simulink model "HQEV_MiL_20160830_integrate_2010a"  (Simulink 7.5)
settings: Solver=FixedStepDiscrete  StartTime=0.0  StopTime=inf  FixedStep=0.01  RelTol=1e-3
PostLoadFcn:
  | , if any(exist('dsrtsu_mdlpostloadfcn', 'file') == [2, 3, 6]), try dsrtsu_mdlpostloadfcn('Execute', bdroot); catch fprintf('Error in PostLoadFcn (dsrtsu_mdlpostloadfcn) for model "%s":\n %s\n', bdroot, lasterr); end, end,
values from neighbouring files (symbols this model uses):
  Bat_C_Ah = 36    [parameter_V1.mat]
  Bat_ocv_xIndex = [5 10 20 30 40 50 60 70 80 90 95]    [parameter_V1.mat]
  Bat_ocv_z = [329 332 340 345 347 351 358 372 377 386 391]    [parameter_V1.mat]
  Bat_R_ohm_z = [4.41 3.46 1.57 1.07 0.76 0.63 0.55 0.44 0.41 0.4 0.4 3.14 ... (66 elements, 11x6)]    [parameter_V1.mat]
  Bat_SOC_Init = 90    [parameter_V1.mat]
  Env_hum_pct_Ambient = 30    [parameter_V1.mat]
  Env_Slope_deg = 0    [parameter_V1.mat]
  Env_Temp_degC_Ambient = 25    [parameter_V1.mat]
  Env_v_kmph_HWind = 0    [parameter_V1.mat]
  Reducer_F_i = 7.23    [parameter_V1.mat]
  Reducer_R_i = 7.23    [parameter_V1.mat]
  Veh =     [parameter_V1.mat]
  Veh_A_m2_Fr = 2.246    [parameter_V1.mat]
  Veh_F_Brake =     [parameter_V1.mat]
  Veh_fac_AirDrag = 0.326    [parameter_V1.mat]
  Veh_fac_WhDragFrict_0 = 0.011    [parameter_V1.mat]
  Veh_g_mps2_C = 9.81    [parameter_V1.mat]
  Veh_GainBrake =     [parameter_V1.mat]
  Veh_h_m_COGHigh = 0.5    [parameter_V1.mat]
  Veh_J_kgm2_Wh = 1.3635    [parameter_V1.mat]
  Veh_L_m_AxlBas = 2.63    [parameter_V1.mat]
  Veh_M_kg = 1427    [parameter_V1.mat]
  Veh_mu_Brake = 0.4    [parameter_V1.mat]
  Veh_mu_Tyre =     [parameter_V1.mat]
  Veh_num_FrictPair = 8    [parameter_V1.mat]
  Veh_pct_Brk = 70    [parameter_V1.mat]
  Veh_r_dyn =     [parameter_V1.mat]
  Veh_r_m_BrkDisk = 0.136    [parameter_V1.mat]
  Veh_rho_kgpm3_Air = 1.2258    [parameter_V1.mat]
undefined symbols (not defined in the file or in its folder): DiscIntNeverNeededParam, p_bool_False_M, p_bool_True_M
libraries: BaseOperationLib_Browser x38, simulink x14, DTQC_lib x1, ERR_lib x1, MQM_lib x1, PTCL_lib x1, PUD_lib x1, TQD_lib x1, TQR_lib x1, VMM_lib x1, ACCA_lib x1, BBCA_lib x1
(part 11 of 15)

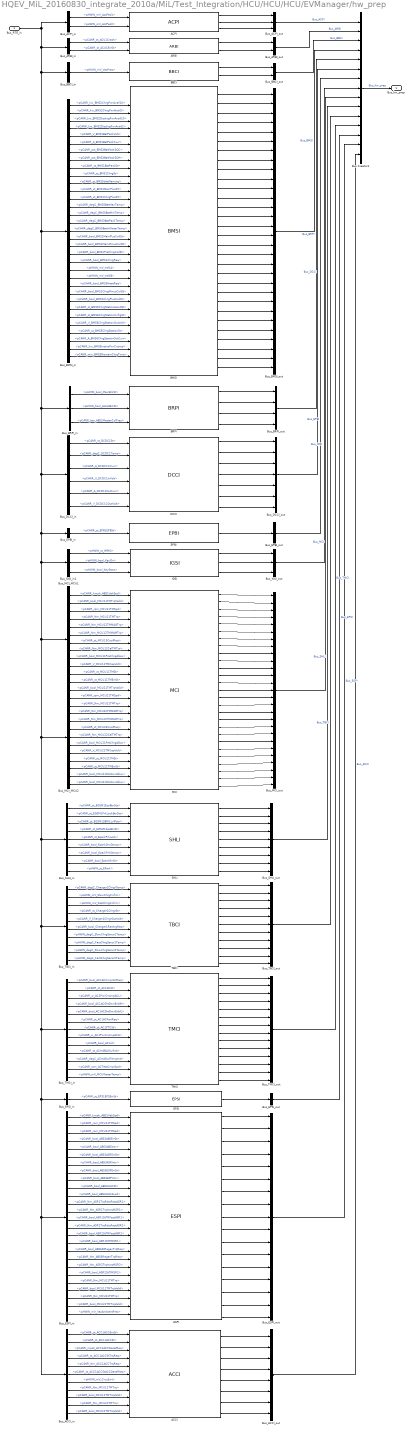
== system HQEV_MiL_20160830_integrate_2010a/MiL/Test_Integration/HCU/HCU/HCU/EVManager/hw_prep ==
  Bus_RTE_in : Inport  OutDataType=fixdt(1, 16)  OutScaling=2^0
  ACCI : ACCI_lib/ACCI  SystemSampleTime=-1
  ACPI : ACPI_lib/ACPI  SystemSampleTime=-1
  ARBI : ARBI_lib/ARBI  SystemSampleTime=-1
  BBCI : BBCI_lib/BBCI  SystemSampleTime=-1
  BMSI : BMSI_lib/BMSI  SystemSampleTime=-1
  BRPI : BRPI_lib/BRPI  SystemSampleTime=-1
  Bus Creator1 : BusCreator  Inputs=15
  Bus_ACCI_in : BusSelector  OutputSignals=pCANR_PT.pCANR_ACC1.pCANR_st_ACC1ACCErrSt,pCANR_PT.pCANR_ACC1.pCANR_st_ACC1ACCSt,pCANR_PT.pCANR_ACC1.pCANR_mps2_ACC1ACCDecelReq,pCANR_PT.pCANR_ACC1.pCANR_st_ACC1ACCStTrqReq,pCANR_PT.pCANR_ACC1.pCANR_Nm_ACC1ACCTrqReq,pCANR_PT.pCANR_ACC1.pCANR_st_ACC1ACCStACCDecelReq,IO.pHWIN_mV_CruzSwt,pCANR_EV.pCANR_MCU.pCANR_MCU1.pCANR_Nm_MCU11TMTrq,pCANR_EV.pCANR_MCU.pCANR_MCU1.pCANR_bool_MCU11TMTrqValid,pCANR_EV.pCANR_MCU.pCANR_MCU1.pCANR_Nm_MCU21TMTrq,pCANR_EV.pCANR_MCU.pCANR_MCU1.pCANR_bool_MCU21TMTrqValid
  Bus_ACCI_out : BusCreator  Inputs=8
  Bus_ACPI_in : BusSelector  OutputSignals=IO.pHWIN_mV_AccPed1,IO.pHWIN_mV_AccPed2
  Bus_ACPI_out : BusCreator  Inputs=3
  Bus_ARBI_in : BusSelector  OutputSignals=pCANR_PT.pCANR_Airbag1.pCANR_st_ACU1Crash,pCANR_PT.pCANR_Airbag1.pCANR_st_ACU1ErrSt
  Bus_ARBI_out : BusCreator  Inputs=2
  Bus_BBCI_in : BusSelector  OutputSignals=IO.pHWIN_mV_VacPres
  Bus_BBCI_out : BusCreator  Inputs=2
  Bus_BMSI_in : BusSelector  OutputSignals=pCANR_EV.pCANR_BMS.pCANR_BMS2.pCANR_kw_BMS2ChrgPwrAvail10,pCANR_EV.pCANR_BMS.pCANR_BMS2.pCANR_kw_BMS2ChrgPwrAvail2,pCANR_EV.pCANR_BMS.pCANR_BMS2.pCANR_kw_BMS2DischrgPwrAvail10,pCANR_EV.pCANR_BMS.pCANR_BMS2.pCANR_kw_BMS2DischrgPwrAvail2,pCANR_EV.pCANR_BMS.pCANR_BMS1.pCANR_V_BMS1BatPackVolt,pCANR_EV.pCANR_BMS.pCANR_BMS1.pCANR_A_BMS1BatPackCurr,pCANR_EV.pCANR_BMS.pCANR_BMS3.pCANR_pct_BMS3BatPackSOC,pCANR_EV.pCANR_BMS.pCANR_BMS3.pCANR_pct_BMS3BatPackSOH,pCANR_EV.pCANR_BMS.pCANR_BMS1.pCANR_st_BMS1BatPackSt,pCANR_EV.pCANR_BMS.pCANR_BMS1.pCANR_st_BMS1ChrgSt,pCANR_EV.pCANR_BMS.pCANR_BMS5.pCANR_st_BMS5IslaWarning,pCANR_EV.pCANR_BMS.pCANR_BMS1.pCANR_st_BMS1MainPlusFlt,pCANR_EV.pCANR_BMS.pCANR_BMS1.pCANR_st_BMS1ChrgPlusFlt,pCANR_EV.pCANR_BMS.pCANR_BMS4.pCANR_degC_BMS5BatMaxTemp,pCANR_EV.pCANR_BMS.pCANR_BMS4.pCANR_degC_BMS5BatMinTemp,pCANR_EV.pCANR_BMS.pCANR_BMS3.pCANR_degC_BMS3BatPackTemp,pCANR_EV.pCANR_BMS.pCANR_BMS4.pCANR_degC_BMS5BatInWaterTemp,pCANR_EV.pCANR_BMS.pCANR_BMS1.pCANR_bool_BMS1MainPlusCoilSt,pCANR_EV.pCANR_BMS.pCANR_BMS1.pCANR_bool_BMS1MainMinusCoilSt,pCANR_EV.pCANR_BMS.pCANR_BMS1.pCANR_bool_BMS1PreChrgCoilSt,pCANR_EV.pCANR_BMS.pCANR_BMS1.pCANR_bool_BMS1ChrgReq,IO.pHWIN_mV_IntlkA,IO.pHWIN_mV_IntlkB,pCANR_EV.pCANR_BMS.pCANR_BMS3.pCANR_bool_BMS3HeatReq,pCANR_EV.pCANR_BMS.pCANR_BMS1.pCANR_bool_BMS1ChrgMinusCoilSt,pCANR_EV.pCANR_BMS.pCANR_BMS1.pCANR_bool_BMS1ChrgPlusCoilSt,pCANR_EV.pCANR_BMS.pCANR_BMS5.pCANR_st_BMS5ChrgStationHandSt,pCANR_EV.pCANR_BMS.pCANR_BMS5.pCANR_st_BMS6ChrgStationCnfigSt,pCANR_EV.pCANR_BMS.pCANR_BMS5.pCANR_V_BMS6ChrgStationOutVolt,pCANR_EV.pCANR_BMS.pCANR_BMS5.pCANR_st_BMS5ChrgStationSt,pCANR_EV.pCANR_BMS.pCANR_BMS5.pCANR_A_BMS6ChrgStationOutCurr,pCANR_EV.pCANR_BMS.pCANR_BMS5.pCANR_kw_BMS6InstnsPwrCnsmp,pCANR_EV.pCANR_BMS.pCANR_BMS5.pCANR_min_BMS5RemainChrgTime
  Bus_BMSI_out : BusCreator  Inputs=30
  Bus_BRPI_in : BusSelector  OutputSignals=IO.pHWIN_bool_MainBrkSt,IO.pHWIN_bool_AssistBrkSt,pCANR_PT.pCANR_ABS.pCANR_ABS2.pCANR_bar_ABS2MasterCylPres
  Bus_BRPI_out : BusCreator
  Bus_DCCI_in : BusSelector  OutputSignals=pCANR_EV.pCANR_DCDC1.pCANR_st_DCDC1St,pCANR_EV.pCANR_DCDC1.pCANR_degC_DCDC1Temp,pCANR_EV.pCANR_DCDC1.pCANR_A_DCDC1InCurr,pCANR_EV.pCANR_DCDC1.pCANR_V_DCDC1InVolt,pCANR_EV.pCANR_DCDC1.pCANR_A_DCDC1OutCurr,pCANR_EV.pCANR_DCDC1.pCANR_V_DCDC1COutVolt
  Bus_DCCI_out : BusCreator  Inputs=7
  Bus_EPBI_in : BusSelector  OutputSignals=pCANR_PT.pCANR_EPB.pCANR_st_EPB1EPBSt
  Bus_EPBI_out : BusCreator  Inputs=1
  Bus_EPSI_in : BusSelector  OutputSignals=pCANR_PT.pCANR_ESP.pCANR_EPS1.pCANR_st_EPS1EPSErrSt
  Bus_EPSI_out : BusCreator  Inputs=1
  Bus_ESPI_in : BusSelector  OutputSignals=pCANR_PT.pCANR_ABS.pCANR_ABS1.pCANR_kmph_ABS1VehSpd,pCANR_EV.pCANR_MCU.pCANR_MCU1.pCANR_rpm_MCU11TMSpd,pCANR_EV.pCANR_MCU.pCANR_MCU1.pCANR_rpm_MCU21TMSpd,pCANR_PT.pCANR_ABS.pCANR_ABS3.pCANR_bool_ABS3ABSErrSt,pCANR_PT.pCANR_ABS.pCANR_ABS3.pCANR_bool_ABS3ABSIntv,pCANR_PT.pCANR_ABS.pCANR_ABS3.pCANR_bool_ABS3ASRErrSt,pCANR_PT.pCANR_ABS.pCANR_ABS3.pCANR_bool_ABS3ASRIntv,pCANR_PT.pCANR_ABS.pCANR_ABS3.pCANR_bool_ABS3ESPErrSt,pCANR_PT.pCANR_ABS.pCANR_ABS3.pCANR_bool_ABS3ESPIntv,pCANR_PT.pCANR_ABS.pCANR_ABS3.pCANR_bool_ABS3HHCSt,pCANR_PT.pCANR_ABS.pCANR_ABS3.pCANR_bool_ABS3HHCAvail,pCANR_PT.pCANR_ASR1.pCANR_Nm_ASR1TrqRdctFastASR1,pCANR_PT.pCANR_ASR1.pCANR_Nm_ASR1TrqIncrsMSR1,pCANR_PT.pCANR_ASR1.pCANR_bool_ASR1StTRFastASR1,pCANR_PT.pCANR_ASR2.pCANR_Nm_ASR2TrqRdctFastASR2,pCANR_PT.pCANR_ASR2.pCANR_bool_ASR2StTRFastASR2,pCANR_PT.pCANR_ASR1.pCANR_bool_ASR1StTIMSR1,pCANR_PT.pCANR_ABS6.pCANR_bool_ABS6StRegenTrqReq,pCANR_PT.pCANR_ABS6.pCANR_Nm_ABS6RegenTrqReq,pCANR_PT.pCANR_ASR2.pCANR_Nm_ASR2TrqIncrsMSR2,pCANR_PT.pCANR_ASR2.pCANR_bool_ASR2StTIMSR2,pCANR_EV.pCANR_MCU.pCANR_MCU1.pCANR_Nm_MCU11TMTrq,pCANR_EV.pCANR_MCU.pCANR_MCU1.pCANR_bool_MCU11TMTrqValid,pCANR_EV.pCANR_MCU.pCANR_MCU1.pCANR_Nm_MCU21TMTrq,pCANR_EV.pCANR_MCU.pCANR_MCU1.pCANR_bool_MCU21TMTrqValid,IO.pHWIN_mV_VacAmbientPres
  Bus_ESPI_out : BusCreator  Inputs=17
  Bus_IGSI_in1 : BusSelector  OutputSignals=IO.pHWIN_st_IMMO,IO.pHWIN_bool_KeyOn,IO.pHWIN_bool_KeyStart
  Bus_IGSI_out : BusCreator  Inputs=3
  Bus_MCI_MCU1 : BusSelector  OutputSignals=pCANR_PT.pCANR_ABS.pCANR_ABS1.pCANR_kmph_ABS1VehSpd,pCANR_EV.pCANR_MCU.pCANR_MCU1.pCANR_bool_MCU11TMTrqValid,pCANR_EV.pCANR_MCU.pCANR_MCU1.pCANR_rpm_MCU11TMSpd,pCANR_EV.pCANR_MCU.pCANR_MCU1.pCANR_Nm_MCU11TMTrq,pCANR_EV.pCANR_MCU.pCANR_MCU2.pCANR_Nm_MCU12TMMAGTrq,pCANR_EV.pCANR_MCU.pCANR_MCU2.pCANR_Nm_MCU12TMMAMTrq,pCANR_EV.pCANR_MCU.pCANR_MCU3.pCANR_st_MCU13CoolReq,pCANR_EV.pCANR_MCU.pCANR_MCU2.pCANR_Nm_MCU12CalTMTrq,pCANR_EV.pCANR_MCU.pCANR_MCU1.pCANR_bool_MCU11PreChrgAllow,pCANR_EV.pCANR_MCU.pCANR_MCU1.pCANR_V_MCU11TMCapVolt,pCANR_EV.pCANR_MCU.pCANR_MCU1.pCANR_st_MCU11TMSt,pCANR_EV.pCANR_MCU.pCANR_MCU1.pCANR_st_MCU11TMErrSt
  Bus_MCI_MCU2 : BusSelector  OutputSignals=pCANR_EV.pCANR_MCU.pCANR_MCU1.pCANR_bool_MCU21TMTrqValid,pCANR_EV.pCANR_MCU.pCANR_MCU1.pCANR_rpm_MCU21TMSpd,pCANR_EV.pCANR_MCU.pCANR_MCU1.pCANR_Nm_MCU21TMTrq,pCANR_EV.pCANR_MCU.pCANR_MCU2.pCANR_Nm_MCU22TMMAGTrq,pCANR_EV.pCANR_MCU.pCANR_MCU2.pCANR_Nm_MCU22TMMAMTrq,pCANR_EV.pCANR_MCU.pCANR_MCU3.pCANR_st_MCU23CoolReq,pCANR_EV.pCANR_MCU.pCANR_MCU2.pCANR_Nm_MCU22CalTMTrq,pCANR_EV.pCANR_MCU.pCANR_MCU1.pCANR_bool_MCU21PreChrgAllow,pCANR_EV.pCANR_MCU.pCANR_MCU1.pCANR_V_MCU21TMCapVolt,pCANR_EV.pCANR_MCU.pCANR_MCU1.pCANR_st_MCU21TMSt,pCANR_EV.pCANR_MCU.pCANR_MCU1.pCANR_st_MCU21TMErrSt,pCANR_EV.pCANR_MCU.pCANR_MCU1.pCANR_bool_MCU11ShtdwnAllow,pCANR_EV.pCANR_MCU.pCANR_MCU1.pCANR_bool_MCU21ShtdwnAllow
  Bus_MCI_out : BusCreator  Inputs=27
  Bus_SHLI_in : BusSelector  OutputSignals=pCANR_PT.pCANR_EGSM1.pCANR_st_EGSM1EcoBtnSts,pCANR_PT.pCANR_EGSM1.pCANR_st_EGSM1PrkLockBtnSts,pCANR_PT.pCANR_EGSM1.pCANR_st_EGSM1SBW1LvlPstn,pCANR_PT.pCANR_EGSM1.pCANR_st_EGSM1SecBtnSt,pCANR_PT.pCAN_ePark_STATE.pCANR_st_EparkPrkLock,pCANR_PT.pCAN_ePark_STATE.pCANR_bool_EparkDrvSensor,pCANR_PT.pCAN_ePark_STATE.pCANR_bool_EparkPrkSensor,pCANR_PT.pCAN_ePark_STATE.pCANR_bool_EparkErrSt,IO.pHWIN_st_EPark
  Bus_SHLI_out : BusCreator  Inputs=9
  Bus_TBCI_in : BusSelector  OutputSignals=pCANR_EV.pCANR_Charger1.pCANR_degC_Charger1ChrgrTemp,IO.pHWIN_mV_SlowChrgCnfrm,IO.pHWIN_mV_FastChrgCnfrm,pCANR_EV.pCANR_Charger1.pCANR_st_Charger1ChrgrSt,pCANR_EV.pCANR_Charger1.pCANR_V_Charger1ChrgrOutVolt,pCANR_EV.pCANR_Charger1.pCANR_bool_Charger1RechrgReq,IO.pHWIN_degC_SlowChrgSensr1Temp,IO.pHWIN_degC_FastChrgSensr1Temp,IO.pHWIN_degC_SlowChrgSensr2Temp,IO.pHWIN_degC_FastChrgSensr2Temp
  Bus_TBCI_out : BusCreator  Inputs=11
  Bus_TMCI_in : BusSelector  OutputSignals=pCANR_PT.pCANR_AC.pCANR_AC1.pCANR_bool_AC1ACCmprOnReq,pCANR_PT.pCANR_AC.pCANR_AC1.pCANR_st_AC1ACSt,pCANR_PT.pCANR_AC.pCANR_AC1.pCANR_w_AC1PwrCnsmpACL,pCANR_PT.pCANR_AC.pCANR_AC1.pCANR_bool_AC1ACShtDwnEnblH,pCANR_PT.pCANR_AC.pCANR_AC1.pCANR_bool_AC1ACShtDwnEnblL,pCANR_PT.pCANR_AC.pCANR_AC1.pCANR_st_AC1ACFanReq,pCANR_PT.pCANR_AC.pCANR_AC1.pCANR_st_AC1PTCSt,pCANR_PT.pCANR_AC.pCANR_AC1.pCANR_w_AC1PwrCnsmpACH,pCANR_PT.pCANR_AC.pCANR_AC1Indication.pCANR_bool_ACInd,pCANR_PT.pCANR_AC.pCANR_AC1Indication.pCANR_st_ACIndBLWLvlInd,pCANR_PT.pCANR_AC.pCANR_AC1Indication.pCANR_degC_ACIndOutTempInd,pCANR_PT.pCANR_AC.pCANR_ACTest.pCANR_rpm_ACTestCmprSpd,IO.pHWIN_mV_MCUWaterTemp
  Bus_TMCI_out : BusCreator  Inputs=14
  DCCI : DCCI_lib/DCCI  SystemSampleTime=-1
  EPBI : EPBI_lib/EPBI  SystemSampleTime=-1
  EPSI : EPSI_lib/EPSI  SystemSampleTime=-1
  ESPI : ESPI_lib/ESPI  SystemSampleTime=-1
  IGSI : IGSI_lib/IGSI  SystemSampleTime=-1
  MCI : MCI_lib/MCI  SystemSampleTime=-1
  SHLI : SHLI_lib/SHLI  SystemSampleTime=-1
  TBCI : TBCI_lib/TBCI  SystemSampleTime=-1
  TMCI : TMCI_lib/TMCI  SystemSampleTime=-1
  Bus_hw_prep : Outport  OutDataType=fixdt(1, 16)  OutScaling=2^0
  wires:
  TBCI/11 -> Bus_TBCI_out/11
  Bus_SHLI_in/8 -> SHLI/8  "<pCANR_bool_EparkErrSt>"
  TBCI/10 -> Bus_TBCI_out/10
  TBCI/9 -> Bus_TBCI_out/9
  TBCI/8 -> Bus_TBCI_out/8
  TBCI/7 -> Bus_TBCI_out/7
  TBCI/6 -> Bus_TBCI_out/6
  TBCI/5 -> Bus_TBCI_out/5
  TBCI/4 -> Bus_TBCI_out/4
  TBCI/3 -> Bus_TBCI_out/3
  TBCI/2 -> Bus_TBCI_out/2
  TBCI/1 -> Bus_TBCI_out/1
  TMCI/14 -> Bus_TMCI_out/14
  TMCI/13 -> Bus_TMCI_out/13
  TMCI/12 -> Bus_TMCI_out/12
  TMCI/11 -> Bus_TMCI_out/11
  TMCI/10 -> Bus_TMCI_out/10
  TMCI/9 -> Bus_TMCI_out/9
  TMCI/8 -> Bus_TMCI_out/8
  TMCI/7 -> Bus_TMCI_out/7
  TMCI/6 -> Bus_TMCI_out/6
  TMCI/5 -> Bus_TMCI_out/5
  TMCI/4 -> Bus_TMCI_out/4
  TMCI/3 -> Bus_TMCI_out/3
  TMCI/2 -> Bus_TMCI_out/2
  TMCI/1 -> Bus_TMCI_out/1
  Bus_TMCI_in/12 -> TMCI/12  "<pCANR_rpm_ACTestCmprSpd>"
  Bus_TMCI_in/13 -> TMCI/13  "<pHWIN_mV_MCUWaterTemp>"
  Bus_TMCI_in/11 -> TMCI/11  "<pCANR_degC_ACIndOutTempInd>"
  Bus_TMCI_in/10 -> TMCI/10  "<pCANR_st_ACIndBLWLvlInd>"
  Bus_TMCI_in/9 -> TMCI/9  "<pCANR_bool_ACInd>"
  Bus_TMCI_in/8 -> TMCI/8  "<pCANR_w_AC1PwrCnsmpACH>"
  Bus_TMCI_in/7 -> TMCI/7  "<pCANR_st_AC1PTCSt>"
  Bus_TMCI_in/6 -> TMCI/6  "<pCANR_st_AC1ACFanReq>"
  Bus_TMCI_in/5 -> TMCI/5  "<pCANR_bool_AC1ACShtDwnEnblL>"
  Bus_TMCI_in/4 -> TMCI/4  "<pCANR_bool_AC1ACShtDwnEnblH>"
  Bus_TMCI_in/3 -> TMCI/3  "<pCANR_w_AC1PwrCnsmpACL>"
  Bus_TMCI_in/2 -> TMCI/2  "<pCANR_st_AC1ACSt>"
  Bus_TMCI_in/1 -> TMCI/1  "<pCANR_bool_AC1ACCmprOnReq>"
  Bus_TMCI_out/1 -> Bus Creator1/12  "Bus_TMCI"
  DCCI/7 -> Bus_DCCI_out/7
  DCCI/6 -> Bus_DCCI_out/6
  DCCI/5 -> Bus_DCCI_out/5
  DCCI/4 -> Bus_DCCI_out/4
  DCCI/3 -> Bus_DCCI_out/3
  DCCI/2 -> Bus_DCCI_out/2
  DCCI/1 -> Bus_DCCI_out/1
  Bus_DCCI_in/6 -> DCCI/6  "<pCANR_V_DCDC1COutVolt>"
  Bus_DCCI_in/5 -> DCCI/5  "<pCANR_A_DCDC1OutCurr>"
  Bus_DCCI_in/4 -> DCCI/4  "<pCANR_V_DCDC1InVolt>"
  Bus_DCCI_in/3 -> DCCI/3  "<pCANR_A_DCDC1InCurr>"
  Bus_DCCI_in/2 -> DCCI/2  "<pCANR_degC_DCDC1Temp>"
  Bus_DCCI_in/1 -> DCCI/1  "<pCANR_st_DCDC1St>"
  Bus_DCCI_out/1 -> Bus Creator1/6  "Bus_DCCI"
  BMSI/30 -> Bus_BMSI_out/30
  BMSI/29 -> Bus_BMSI_out/29
  BMSI/28 -> Bus_BMSI_out/28
  BMSI/27 -> Bus_BMSI_out/27
  BMSI/26 -> Bus_BMSI_out/26
  BMSI/25 -> Bus_BMSI_out/25
  BMSI/24 -> Bus_BMSI_out/24
  BMSI/23 -> Bus_BMSI_out/23
  BMSI/22 -> Bus_BMSI_out/22
  BMSI/21 -> Bus_BMSI_out/21
  BMSI/20 -> Bus_BMSI_out/20
  BMSI/19 -> Bus_BMSI_out/19
  BMSI/18 -> Bus_BMSI_out/18
  BMSI/17 -> Bus_BMSI_out/17
  BMSI/16 -> Bus_BMSI_out/16
  BMSI/15 -> Bus_BMSI_out/15
  BMSI/14 -> Bus_BMSI_out/14
  BMSI/13 -> Bus_BMSI_out/13
  BMSI/12 -> Bus_BMSI_out/12
  Bus_SHLI_in/9 -> SHLI/9  "<pHWIN_st_EPark>"
  SHLI/9 -> Bus_SHLI_out/9
  SHLI/8 -> Bus_SHLI_out/8
  SHLI/7 -> Bus_SHLI_out/7
  SHLI/6 -> Bus_SHLI_out/6
  SHLI/5 -> Bus_SHLI_out/5
  SHLI/4 -> Bus_SHLI_out/4
  SHLI/3 -> Bus_SHLI_out/3
  SHLI/2 -> Bus_SHLI_out/2
  SHLI/1 -> Bus_SHLI_out/1
  Bus_SHLI_in/4 -> SHLI/4  "<pCANR_st_EGSM1SecBtnSt>"
  Bus_SHLI_in/7 -> SHLI/7  "<pCANR_bool_EparkPrkSensor>"
  Bus_SHLI_in/6 -> SHLI/6  "<pCANR_bool_EparkDrvSensor>"
  Bus_SHLI_in/5 -> SHLI/5  "<pCANR_st_EparkPrkLock>"
  Bus_SHLI_in/3 -> SHLI/3  "<pCANR_st_EGSM1SBW1LvlPstn>"
  Bus_SHLI_in/2 -> SHLI/2  "<pCANR_st_EGSM1PrkLockBtnSts>"
  Bus_SHLI_in/1 -> SHLI/1  "<pCANR_st_EGSM1EcoBtnSts>"
  BMSI/11 -> Bus_BMSI_out/11
  BMSI/10 -> Bus_BMSI_out/10
  BMSI/9 -> Bus_BMSI_out/9
  BMSI/8 -> Bus_BMSI_out/8
  BMSI/7 -> Bus_BMSI_out/7
  BMSI/6 -> Bus_BMSI_out/6
  BMSI/5 -> Bus_BMSI_out/5
  BMSI/4 -> Bus_BMSI_out/4
  BMSI/3 -> Bus_BMSI_out/3
  BMSI/2 -> Bus_BMSI_out/2
  BMSI/1 -> Bus_BMSI_out/1
  Bus_BMSI_in/13 -> BMSI/13  "<pCANR_st_BMS1ChrgPlusFlt>"
  Bus_BMSI_in/12 -> BMSI/12  "<pCANR_st_BMS1MainPlusFlt>"
  Bus_BMSI_in/33 -> BMSI/33  "<pCANR_min_BMS5RemainChrgTime>"
  Bus_ESPI_out/1 -> Bus Creator1/14  "Bus_ESPI"
  Bus_BMSI_in/32 -> BMSI/32  "<pCANR_kw_BMS6InstnsPwrCnsmp>"
  Bus_TBCI_in/10 -> TBCI/10  "<pHWIN_degC_FastChrgSensr2Temp>"
  Bus_TBCI_in/9 -> TBCI/9  "<pHWIN_degC_SlowChrgSensr2Temp>"
  Bus_TBCI_in/8 -> TBCI/8  "<pHWIN_degC_FastChrgSensr1Temp>"
  Bus_TBCI_in/7 -> TBCI/7  "<pHWIN_degC_SlowChrgSensr1Temp>"
  Bus_BMSI_in/1 -> BMSI/1  "<pCANR_kw_BMS2ChrgPwrAvail10>"
  Bus_IGSI_in1/3 -> IGSI/3  "<pHWIN_bool_KeyStart>"
  Bus_IGSI_in1/2 -> IGSI/2  "<pHWIN_bool_KeyOn>"
  Bus_IGSI_in1/1 -> IGSI/1  "<pHWIN_st_IMMO>"
  Bus_BMSI_in/31 -> BMSI/31  "<pCANR_A_BMS6ChrgStationOutCurr>"
  Bus_BMSI_in/30 -> BMSI/30  "<pCANR_st_BMS5ChrgStationSt>"
  Bus_BMSI_in/29 -> BMSI/29  "<pCANR_V_BMS6ChrgStationOutVolt>"
  Bus_BMSI_in/28 -> BMSI/28  "<pCANR_st_BMS6ChrgStationCnfigSt>"
  Bus_BMSI_in/27 -> BMSI/27  "<pCANR_st_BMS5ChrgStationHandSt>"
  Bus_BMSI_in/26 -> BMSI/26  "<pCANR_bool_BMS1ChrgPlusCoilSt>"
  Bus_BMSI_in/25 -> BMSI/25  "<pCANR_bool_BMS1ChrgMinusCoilSt>"
  Bus_BMSI_in/24 -> BMSI/24  "<pCANR_bool_BMS3HeatReq>"
  Bus_BMSI_in/23 -> BMSI/23  "<pHWIN_mV_IntlkB>"
  Bus_BMSI_in/22 -> BMSI/22  "<pHWIN_mV_IntlkA>"
  Bus_BMSI_in/21 -> BMSI/21  "<pCANR_bool_BMS1ChrgReq>"
  Bus_BMSI_in/20 -> BMSI/20  "<pCANR_bool_BMS1PreChrgCoilSt>"
  Bus_BMSI_in/19 -> BMSI/19  "<pCANR_bool_BMS1MainMinusCoilSt>"
  Bus_BMSI_in/18 -> BMSI/18  "<pCANR_bool_BMS1MainPlusCoilSt>"
  Bus_BMSI_in/17 -> BMSI/17  "<pCANR_degC_BMS5BatInWaterTemp>"
  Bus_BMSI_in/16 -> BMSI/16  "<pCANR_degC_BMS3BatPackTemp>"
  Bus_BMSI_in/15 -> BMSI/15  "<pCANR_degC_BMS5BatMinTemp>"
  Bus_BMSI_in/14 -> BMSI/14  "<pCANR_degC_BMS5BatMaxTemp>"
  Bus_BMSI_in/11 -> BMSI/11  "<pCANR_st_BMS5IslaWarning>"
  Bus_BMSI_in/10 -> BMSI/10  "<pCANR_st_BMS1ChrgSt>"
  Bus_BMSI_in/9 -> BMSI/9  "<pCANR_st_BMS1BatPackSt>"
  Bus_BMSI_in/8 -> BMSI/8  "<pCANR_pct_BMS3BatPackSOH>"
  Bus_BMSI_in/7 -> BMSI/7  "<pCANR_pct_BMS3BatPackSOC>"
  Bus_BMSI_in/6 -> BMSI/6  "<pCANR_A_BMS1BatPackCurr>"
  Bus_BMSI_in/5 -> BMSI/5  "<pCANR_V_BMS1BatPackVolt>"
  Bus_BMSI_in/4 -> BMSI/4  "<pCANR_kw_BMS2DischrgPwrAvail2>"
  Bus_BMSI_in/3 -> BMSI/3  "<pCANR_kw_BMS2DischrgPwrAvail10>"
  Bus_BMSI_in/2 -> BMSI/2  "<pCANR_kw_BMS2ChrgPwrAvail2>"
  IGSI/2 -> Bus_IGSI_out/2
  IGSI/1 -> Bus_IGSI_out/1
  BRPI/2 -> Bus_BRPI_out/2
  BRPI/1 -> Bus_BRPI_out/1
  Bus_BRPI_in/3 -> BRPI/3  "<pCANR_bar_ABS2MasterCylPres>"
  Bus_BRPI_in/2 -> BRPI/2  "<pHWIN_bool_AssistBrkSt>"
  BBCI/2 -> Bus_BBCI_out/2
  BBCI/1 -> Bus_BBCI_out/1
  ACPI/2 -> Bus_ACPI_out/2
  ACPI/1 -> Bus_ACPI_out/1
  Bus_TBCI_out/1 -> Bus Creator1/11  "Bus_TBCI"
  Bus_SHLI_out/1 -> Bus Creator1/10  "Bus_SHLI"
  Bus_IGSI_out/1 -> Bus Creator1/8  "Bus_IGSI"
  Bus_EPBI_out/1 -> Bus Creator1/7  "Bus_EPBI"
  Bus_BRPI_out/1 -> Bus Creator1/5  "Bus_BRPI"
  Bus_BMSI_out/1 -> Bus Creator1/4  "Bus_BMSI"
  Bus_BBCI_out/1 -> Bus Creator1/3  "Bus_BBCI"
  Bus_ARBI_out/1 -> Bus Creator1/2  "Bus_ARBI"
  Bus_ACPI_out/1 -> Bus Creator1/1  "Bus_ACPI"
  ARBI/1 -> Bus_ARBI_out/1
  Bus_ARBI_in/1 -> ARBI/1  "<pCANR_st_ACU1Crash>"
  Bus_ACPI_in/2 -> ACPI/2  "<pHWIN_mV_AccPed2>"
  Bus_ACPI_in/1 -> ACPI/1  "<pHWIN_mV_AccPed1>"
  EPBI/1 -> Bus_EPBI_out/1
  Bus_EPBI_in/1 -> EPBI/1  "<pCANR_st_EPB1EPBSt>"
  Bus_BBCI_in/1 -> BBCI/1  "<pHWIN_mV_VacPres>"
  Bus_RTE_in/1 -> Bus_ACPI_in/1, Bus_BMSI_in/1, Bus_DCCI_in/1, Bus_MCI_MCU1/1, Bus_TMCI_in/1, Bus_EPSI_in/1, Bus_ESPI_in/1, Bus_ACCI_in/1, Bus_TBCI_in/1, Bus_SHLI_in/1, Bus_MCI_MCU2/1, Bus_IGSI_in1/1, Bus_EPBI_in/1, Bus_BRPI_in/1, Bus_BBCI_in/1, Bus_ARBI_in/1
  Bus Creator1/1 -> Bus_hw_prep/1  "Bus_hw_prep"
  BRPI/3 -> Bus_BRPI_out/3
  Bus_BRPI_in/1 -> BRPI/1  "<pHWIN_bool_MainBrkSt>"
  Bus_ARBI_in/2 -> ARBI/2  "<pCANR_st_ACU1ErrSt>"
  ARBI/2 -> Bus_ARBI_out/2
  BRPI/4 -> Bus_BRPI_out/4
  IGSI/3 -> Bus_IGSI_out/3
  Bus_EPSI_in/1 -> EPSI/1  "<pCANR_st_EPS1EPSErrSt>"
  EPSI/1 -> Bus_EPSI_out/1
  Bus_EPSI_out/1 -> Bus Creator1/13  "Bus_EPSI"
  Bus_TBCI_in/1 -> TBCI/1  "<pCANR_degC_Charger1ChrgrTemp>"
  Bus_TBCI_in/2 -> TBCI/2  "<pHWIN_mV_SlowChrgCnfrm>"
  Bus_TBCI_in/4 -> TBCI/4  "<pCANR_st_Charger1ChrgrSt>"
  Bus_TBCI_in/5 -> TBCI/5  "<pCANR_V_Charger1ChrgrOutVolt>"
  Bus_TBCI_in/6 -> TBCI/6  "<pCANR_bool_Charger1RechrgReq>"
  Bus_TBCI_in/3 -> TBCI/3  "<pHWIN_mV_FastChrgCnfrm>"
  ACCI/1 -> Bus_ACCI_out/1
  ACCI/2 -> Bus_ACCI_out/2
  ACCI/3 -> Bus_ACCI_out/3
  ACCI/4 -> Bus_ACCI_out/4
  ACCI/5 -> Bus_ACCI_out/5
  ACCI/6 -> Bus_ACCI_out/6
  Bus_ACCI_out/1 -> Bus Creator1/15  "Bus_ACCI"
  Bus_ACCI_in/1 -> ACCI/1  "<pCANR_st_ACC1ACCErrSt>"
  Bus_ACCI_in/2 -> ACCI/2  "<pCANR_st_ACC1ACCSt>"
  Bus_ACCI_in/4 -> ACCI/4  "<pCANR_st_ACC1ACCStTrqReq>"
  Bus_ACCI_in/5 -> ACCI/5  "<pCANR_Nm_ACC1ACCTrqReq>"
  Bus_ACCI_in/6 -> ACCI/6  "<pCANR_st_ACC1ACCStACCDecelReq>"
  Bus_ACCI_in/7 -> ACCI/7  "<pHWIN_mV_CruzSwt>"
  Bus_ACCI_in/8 -> ACCI/8  "<pCANR_Nm_MCU11TMTrq>"
  Bus_ACCI_in/9 -> ACCI/9  "<pCANR_bool_MCU11TMTrqValid>"
  Bus_ACCI_in/10 -> ACCI/10  "<pCANR_Nm_MCU21TMTrq>"
  Bus_ACCI_in/11 -> ACCI/11  "<pCANR_bool_MCU21TMTrqValid>"
  ACCI/7 -> Bus_ACCI_out/7
  ACCI/8 -> Bus_ACCI_out/8
  ESPI/1 -> Bus_ESPI_out/1
  ESPI/2 -> Bus_ESPI_out/2
  ESPI/3 -> Bus_ESPI_out/3
  ESPI/4 -> Bus_ESPI_out/4
  ESPI/5 -> Bus_ESPI_out/5
  ESPI/6 -> Bus_ESPI_out/6
  ESPI/7 -> Bus_ESPI_out/7
  ESPI/8 -> Bus_ESPI_out/8
  ESPI/9 -> Bus_ESPI_out/9
  ESPI/10 -> Bus_ESPI_out/10
  ESPI/11 -> Bus_ESPI_out/11
  ESPI/12 -> Bus_ESPI_out/12
  ESPI/13 -> Bus_ESPI_out/13
  ESPI/14 -> Bus_ESPI_out/14
  ESPI/15 -> Bus_ESPI_out/15
  ESPI/16 -> Bus_ESPI_out/16
  Bus_ESPI_in/1 -> ESPI/1  "<pCANR_kmph_ABS1VehSpd>"
  Bus_ESPI_in/2 -> ESPI/2  "<pCANR_rpm_MCU11TMSpd>"
  Bus_ESPI_in/3 -> ESPI/3  "<pCANR_rpm_MCU21TMSpd>"
  Bus_ESPI_in/4 -> ESPI/4  "<pCANR_bool_ABS3ABSErrSt>"
  Bus_ESPI_in/5 -> ESPI/5  "<pCANR_bool_ABS3ABSIntv>"
  Bus_ESPI_in/6 -> ESPI/6  "<pCANR_bool_ABS3ASRErrSt>"
  Bus_ESPI_in/7 -> ESPI/7  "<pCANR_bool_ABS3ASRIntv>"
  Bus_ESPI_in/8 -> ESPI/8  "<pCANR_bool_ABS3ESPErrSt>"
  Bus_ESPI_in/9 -> ESPI/9  "<pCANR_bool_ABS3ESPIntv>"
  Bus_ESPI_in/10 -> ESPI/10  "<pCANR_bool_ABS3HHCSt>"
  Bus_ESPI_in/11 -> ESPI/11  "<pCANR_bool_ABS3HHCAvail>"
  Bus_ESPI_in/12 -> ESPI/12  "<pCANR_Nm_ASR1TrqRdctFastASR1>"
  Bus_ESPI_in/13 -> ESPI/13  "<pCANR_Nm_ASR1TrqIncrsMSR1>"
  Bus_ESPI_in/14 -> ESPI/14  "<pCANR_bool_ASR1StTRFastASR1>"
  Bus_ESPI_in/15 -> ESPI/15  "<pCANR_Nm_ASR2TrqRdctFastASR2>"
  Bus_ESPI_in/16 -> ESPI/16  "<pCANR_bool_ASR2StTRFastASR2>"
  Bus_ESPI_in/17 -> ESPI/17  "<pCANR_bool_ASR1StTIMSR1>"
  Bus_ESPI_in/18 -> ESPI/18  "<pCANR_bool_ABS6StRegenTrqReq>"
  Bus_ESPI_in/19 -> ESPI/19  "<pCANR_Nm_ABS6RegenTrqReq>"
  Bus_ESPI_in/20 -> ESPI/20  "<pCANR_Nm_ASR2TrqIncrsMSR2>"
  Bus_ESPI_in/21 -> ESPI/21  "<pCANR_bool_ASR2StTIMSR2>"
  Bus_ESPI_in/22 -> ESPI/22  "<pCANR_Nm_MCU11TMTrq>"
  Bus_ESPI_in/23 -> ESPI/23  "<pCANR_bool_MCU11TMTrqValid>"
  Bus_ESPI_in/24 -> ESPI/24  "<pCANR_Nm_MCU21TMTrq>"
  Bus_ESPI_in/25 -> ESPI/25  "<pCANR_bool_MCU21TMTrqValid>"
  Bus_ACCI_in/3 -> ACCI/3  "<pCANR_mps2_ACC1ACCDecelReq>"
  Bus_MCI_MCU2/1 -> MCI/13  "<pCANR_bool_MCU21TMTrqValid>"
  Bus_MCI_MCU1/2 -> MCI/2  "<pCANR_bool_MCU11TMTrqValid>"
  Bus_MCI_MCU2/11 -> MCI/23  "<pCANR_st_MCU21TMErrSt>"
  Bus_MCI_MCU2/10 -> MCI/22  "<pCANR_st_MCU21TMSt>"
  Bus_MCI_MCU2/9 -> MCI/21  "<pCANR_V_MCU21TMCapVolt>"
  Bus_MCI_MCU2/8 -> MCI/20  "<pCANR_bool_MCU21PreChrgAllow>"
  Bus_MCI_MCU2/7 -> MCI/19  "<pCANR_Nm_MCU22CalTMTrq>"
  Bus_MCI_MCU2/6 -> MCI/18  "<pCANR_st_MCU23CoolReq>"
  Bus_MCI_MCU2/5 -> MCI/17  "<pCANR_Nm_MCU22TMMAMTrq>"
  Bus_MCI_MCU2/4 -> MCI/16  "<pCANR_Nm_MCU22TMMAGTrq>"
  Bus_MCI_MCU2/3 -> MCI/15  "<pCANR_Nm_MCU21TMTrq>"
  Bus_MCI_MCU2/2 -> MCI/14  "<pCANR_rpm_MCU21TMSpd>"
  Bus_MCI_MCU1/12 -> MCI/12  "<pCANR_st_MCU11TMErrSt>"
  Bus_MCI_MCU1/11 -> MCI/11  "<pCANR_st_MCU11TMSt>"
  Bus_MCI_MCU1/10 -> MCI/10  "<pCANR_V_MCU11TMCapVolt>"
  Bus_MCI_MCU1/9 -> MCI/9  "<pCANR_bool_MCU11PreChrgAllow>"
  Bus_MCI_MCU1/8 -> MCI/8  "<pCANR_Nm_MCU12CalTMTrq>"
  Bus_MCI_MCU1/7 -> MCI/7  "<pCANR_st_MCU13CoolReq>"
  Bus_MCI_MCU1/6 -> MCI/6  "<pCANR_Nm_MCU12TMMAMTrq>"
  Bus_MCI_MCU1/5 -> MCI/5  "<pCANR_Nm_MCU12TMMAGTrq>"
  Bus_MCI_MCU1/4 -> MCI/4  "<pCANR_Nm_MCU11TMTrq>"
  Bus_MCI_MCU1/3 -> MCI/3  "<pCANR_rpm_MCU11TMSpd>"
  Bus_MCI_MCU1/1 -> MCI/1  "<pCANR_kmph_ABS1VehSpd>"
  Bus_MCI_out/1 -> Bus Creator1/9  "Bus_MCI"
  Bus_MCI_MCU2/12 -> MCI/24  "<pCANR_bool_MCU11ShtdwnAllow>"
  Bus_MCI_MCU2/13 -> MCI/25  "<pCANR_bool_MCU21ShtdwnAllow>"
  MCI/1 -> Bus_MCI_out/1
  MCI/2 -> Bus_MCI_out/2
  MCI/3 -> Bus_MCI_out/3
  MCI/4 -> Bus_MCI_out/4
  MCI/5 -> Bus_MCI_out/5
  MCI/6 -> Bus_MCI_out/6
  MCI/7 -> Bus_MCI_out/7
  MCI/8 -> Bus_MCI_out/8
  MCI/9 -> Bus_MCI_out/9
  MCI/10 -> Bus_MCI_out/10
  MCI/11 -> Bus_MCI_out/11
  MCI/12 -> Bus_MCI_out/12
  MCI/13 -> Bus_MCI_out/13
  MCI/14 -> Bus_MCI_out/14
  MCI/15 -> Bus_MCI_out/15
  MCI/16 -> Bus_MCI_out/16
  MCI/17 -> Bus_MCI_out/17
  MCI/18 -> Bus_MCI_out/18
  MCI/19 -> Bus_MCI_out/19
  MCI/20 -> Bus_MCI_out/20
  MCI/21 -> Bus_MCI_out/21
  MCI/22 -> Bus_MCI_out/22
  MCI/23 -> Bus_MCI_out/23
  MCI/24 -> Bus_MCI_out/24
  MCI/25 -> Bus_MCI_out/25
  MCI/26 -> Bus_MCI_out/26
  MCI/27 -> Bus_MCI_out/27
  ACPI/3 -> Bus_ACPI_out/3
  Bus_ESPI_in/26 -> ESPI/26  "<pHWIN_mV_VacAmbientPres>"
  ESPI/17 -> Bus_ESPI_out/17

== system HQEV_MiL_20160830_integrate_2010a/MiL/Test_Integration/MCU_FF/MCU/MCU/GSD/Subsystem ==
  In1 : Inport
  Constant11 : Constant
  Constant2 : Constant  Value=5
  Ground{,1..4,6..12} (12 alike) : Ground
  Terminator : Terminator
  MCU1_TMSpeed : Outport
  MCU1_ActTMTorque : Outport  Port=2
  MCU1_TMCapacitanceVoltage : Outport  Port=3
  MCU1_ActualTMTorqueValid : Outport  Port=4
  MCU1_MCU1 PrechargeAllow : Outport  Port=5
  MCU1_TMStatus : Outport  Port=6
  MCU1_TMErrorStatus : Outport  Port=7
  MCU1_TM MAMTorque : Outport  Port=8
  MCU1_TM MAGTorque : Outport  Port=9
  MCU1_CalTMTorque : Outport  Port=10
  MCU1_CoolingRequest : Outport  Port=11
  PWM_Status : Outport  Port=12
  EM_trq_req : Outport  Port=13
  bool_MCUPwrDwnAllow : Outport  Port=14
  wires:
  Ground/1 -> MCU1_TMSpeed/1
  Ground1/1 -> MCU1_ActTMTorque/1
  Ground2/1 -> MCU1_TMCapacitanceVoltage/1
  Ground3/1 -> MCU1_ActualTMTorqueValid/1
  Ground4/1 -> MCU1_MCU1 PrechargeAllow/1
  Constant2/1 -> MCU1_TMStatus/1
  Ground6/1 -> MCU1_TMErrorStatus/1
  Ground7/1 -> MCU1_TM MAMTorque/1
  Ground8/1 -> MCU1_TM MAGTorque/1
  Ground9/1 -> MCU1_CalTMTorque/1
  Ground10/1 -> MCU1_CoolingRequest/1
  Ground11/1 -> PWM_Status/1
  Ground12/1 -> EM_trq_req/1
  In1/1 -> Terminator/1
  Constant11/1 -> bool_MCUPwrDwnAllow/1

== system HQEV_MiL_20160830_integrate_2010a/MiL/Test_Integration/MCU_FF/MCU/MCU/Init/Subsystem ==
  In1 : Inport
  Bus Selector : BusSelector  OutputSignals=Motor_F.EM1_spd
  Bus Selector1 : BusSelector  OutputSignals=Motor_F.EM1_U
  Constant{,1..10} (11 alike) : Constant  Value=0
  Constant11 : Constant
  Unit Delay : UnitDelay  SampleTime=-1
  Unit Delay1 : UnitDelay  SampleTime=-1
  MCU1_TMSpeed : Outport
  MCU1_ActTMTorque : Outport  Port=2
  MCU1_TMCapacitanceVoltage : Outport  Port=3
  MCU1_ActualTMTorqueValid : Outport  Port=4
  MCU1_MCU1PrechargeAllow : Outport  Port=5
  MCU1_TMStatus : Outport  Port=6
  MCU1_TMErrorStatus : Outport  Port=7
  MCU1_TM MAMTorque : Outport  Port=8
  MCU1_TM MAGTorque : Outport  Port=9
  MCU1_CalTMTorque : Outport  Port=10
  MCU1_CoolingRequest : Outport  Port=11
  PWM_Status : Outport  Port=12
  EM_trq_req : Outport  Port=13
  bool_MCUPwrDwnAllow : Outport  Port=14
  wires:
  Constant/1 -> MCU1_ActualTMTorqueValid/1
  Constant1/1 -> MCU1_MCU1PrechargeAllow/1
  Constant2/1 -> MCU1_TMStatus/1
  Constant3/1 -> MCU1_TMErrorStatus/1
  Constant4/1 -> MCU1_TM MAMTorque/1
  Constant5/1 -> MCU1_TM MAGTorque/1
  Constant6/1 -> MCU1_CalTMTorque/1
  Constant7/1 -> MCU1_CoolingRequest/1
  Constant8/1 -> PWM_Status/1
  Constant9/1 -> EM_trq_req/1
  Constant10/1 -> MCU1_ActTMTorque/1
  Bus Selector/1 -> Unit Delay/1  "<EM1_spd>"
  Bus Selector1/1 -> Unit Delay1/1  "<EM1_U>"
  In1/1 -> Bus Selector/1, Bus Selector1/1
  Unit Delay/1 -> MCU1_TMSpeed/1
  Unit Delay1/1 -> MCU1_TMCapacitanceVoltage/1
  Constant11/1 -> bool_MCUPwrDwnAllow/1

== system HQEV_MiL_20160830_integrate_2010a/MiL/Test_Integration/MCU_FF/MCU/MCU/Invalid/Subsystem ==
  In1 : Inport
  Constant11 : Constant
  Ground{,1..12} (13 alike) : Ground
  Terminator : Terminator
  MCU1_TMSpeed : Outport
  MCU1_ActTMTorque : Outport  Port=2
  MCU1_TMCapacitanceVoltage : Outport  Port=3
  MCU1_ActualTMTorqueValid : Outport  Port=4
  MCU1_MCU1 PrechargeAllow : Outport  Port=5
  MCU1_TMStatus : Outport  Port=6
  MCU1_TMErrorStatus : Outport  Port=7
  MCU1_TM MAMTorque : Outport  Port=8
  MCU1_TM MAGTorque : Outport  Port=9
  MCU1_CalTMTorque : Outport  Port=10
  MCU1_CoolingRequest : Outport  Port=11
  PWM_Status : Outport  Port=12
  EM_trq_req : Outport  Port=13
  bool_MCUPwrDwnAllow : Outport  Port=14
  wires:
  Ground/1 -> MCU1_TMSpeed/1
  Ground1/1 -> MCU1_ActTMTorque/1
  Ground2/1 -> MCU1_TMCapacitanceVoltage/1
  Ground3/1 -> MCU1_ActualTMTorqueValid/1
  Ground4/1 -> MCU1_MCU1 PrechargeAllow/1
  Ground5/1 -> MCU1_TMStatus/1
  Ground6/1 -> MCU1_TMErrorStatus/1
  Ground7/1 -> MCU1_TM MAMTorque/1
  Ground8/1 -> MCU1_TM MAGTorque/1
  Ground9/1 -> MCU1_CalTMTorque/1
  Ground10/1 -> MCU1_CoolingRequest/1
  Ground11/1 -> PWM_Status/1
  Ground12/1 -> EM_trq_req/1
  In1/1 -> Terminator/1
  Constant11/1 -> bool_MCUPwrDwnAllow/1

== system HQEV_MiL_20160830_integrate_2010a/MiL/Test_Integration/MCU_FF/MCU/MCU/Precharge/Subsystem ==
  In1 : Inport
  Bus Selector : BusSelector  OutputSignals=Motor_F.EM1_spd
  Bus Selector1 : BusSelector  OutputSignals=Motor_F.EM1_U
  Constant{,3..10} (9 alike) : Constant  Value=0
  Constant1 : Constant
  Constant11 : Constant
  Constant2 : Constant
  Unit Delay : UnitDelay  SampleTime=-1
  Unit Delay1 : UnitDelay  SampleTime=-1
  MCU1_TMSpeed : Outport
  MCU1_ActTMTorque : Outport  Port=2
  MCU1_TMCapacitanceVoltage : Outport  Port=3
  MCU1_ActualTMTorqueValid : Outport  Port=4
  MCU1_MCU1 PrechargeAllow : Outport  Port=5
  MCU1_TMStatus : Outport  Port=6
  MCU1_TMErrorStatus : Outport  Port=7
  MCU1_TM MAMTorque : Outport  Port=8
  MCU1_TM MAGTorque : Outport  Port=9
  MCU1_CalTMTorque : Outport  Port=10
  MCU1_CoolingRequest : Outport  Port=11
  PWM_Status : Outport  Port=12
  EM_trq_req : Outport  Port=13
  bool_MCUPwrDwnAllow : Outport  Port=14
  wires:
  Constant10/1 -> MCU1_ActTMTorque/1
  Constant/1 -> MCU1_ActualTMTorqueValid/1
  Constant1/1 -> MCU1_MCU1 PrechargeAllow/1
  Constant2/1 -> MCU1_TMStatus/1
  Constant3/1 -> MCU1_TMErrorStatus/1
  Constant4/1 -> MCU1_TM MAMTorque/1
  Constant5/1 -> MCU1_TM MAGTorque/1
  Constant6/1 -> MCU1_CalTMTorque/1
  Constant7/1 -> MCU1_CoolingRequest/1
  Constant8/1 -> PWM_Status/1
  Constant9/1 -> EM_trq_req/1
  Bus Selector/1 -> Unit Delay/1  "<EM1_spd>"
  Bus Selector1/1 -> Unit Delay1/1  "<EM1_U>"
  In1/1 -> Bus Selector/1, Bus Selector1/1
  Unit Delay/1 -> MCU1_TMSpeed/1
  Unit Delay1/1 -> MCU1_TMCapacitanceVoltage/1
  Constant11/1 -> bool_MCUPwrDwnAllow/1

== system HQEV_MiL_20160830_integrate_2010a/MiL/Test_Integration/MCU_FF/MCU/MCU/Rapid_Discharge/Subsystem ==
  In1 : Inport
  Bus Selector : BusSelector  OutputSignals=Motor_F.EM1_spd
  Bus Selector1 : BusSelector  OutputSignals=Motor_F.EM1_U
  Constant{,1..2,4..9} (9 alike) : Constant  Value=0
  Constant11 : Constant
  Constant3 : Constant  Value=6
  Subsystem : Subsystem
  Unit Delay : UnitDelay  SampleTime=-1
  Unit Delay1 : UnitDelay  SampleTime=-1
  MCU1_TMSpeed : Outport
  MCU1_ActTMTorque : Outport  Port=2
  MCU1_TMCapacitanceVoltage : Outport  Port=3
  MCU1_ActualTMTorqueValid : Outport  Port=4
  MCU1_MCU1 PrechargeAllow : Outport  Port=5
  MCU1_TMStatus : Outport  Port=6
  MCU1_TMErrorStatus : Outport  Port=7
  MCU1_TM MAMTorque : Outport  Port=8
  MCU1_TM MAGTorque : Outport  Port=9
  MCU1_CalTMTorque : Outport  Port=10
  MCU1_CoolingRequest : Outport  Port=11
  PWM_Status : Outport  Port=12
  EM_trq_req : Outport  Port=13
  bool_MCUPwrDwnAllow : Outport  Port=14
  wires:
  Constant/1 -> MCU1_ActTMTorque/1
  Constant1/1 -> MCU1_ActualTMTorqueValid/1
  Constant2/1 -> MCU1_MCU1 PrechargeAllow/1
  Constant3/1 -> MCU1_TMStatus/1
  Constant4/1 -> MCU1_TMErrorStatus/1
  Constant5/1 -> MCU1_TM MAMTorque/1
  Constant6/1 -> MCU1_TM MAGTorque/1
  Constant7/1 -> MCU1_CalTMTorque/1
  Constant8/1 -> MCU1_CoolingRequest/1
  Subsystem/1(PWM) -> PWM_Status/1
  Constant9/1 -> EM_trq_req/1
  In1/1 -> Bus Selector/1, Bus Selector1/1
  Bus Selector/1 -> Unit Delay/1  "<EM1_spd>"
  Bus Selector1/1 -> Unit Delay1/1  "<EM1_U>"
  Unit Delay/1 -> Subsystem/1(EM_spd), MCU1_TMSpeed/1
  Unit Delay1/1 -> MCU1_TMCapacitanceVoltage/1
  Constant11/1 -> bool_MCUPwrDwnAllow/1

== system HQEV_MiL_20160830_integrate_2010a/MiL/Test_Integration/MCU_FF/MCU/MCU/Sleep/Subsystem ==
  In1 : Inport
  Constant : Constant  Value=0
  Constant11 : Constant
  Ground{,1..4,6..12} (12 alike) : Ground
  Terminator : Terminator
  MCU1_TMSpeed : Outport
  MCU1_ActTMTorque : Outport  Port=2
  MCU1_TMCapacitanceVoltage : Outport  Port=3
  MCU1_ActualTMTorqueValid : Outport  Port=4
  MCU1_MCU1 PrechargeAllow : Outport  Port=5
  MCU1_TMStatus : Outport  Port=6
  MCU1_TMErrorStatus : Outport  Port=7
  MCU1_TM MAMTorque : Outport  Port=8
  MCU1_TM MAGTorque : Outport  Port=9
  MCU1_CalTMTorque : Outport  Port=10
  MCU1_CoolingRequest : Outport  Port=11
  PWM_Status : Outport  Port=12
  EM_trq_req : Outport  Port=13
  bool_MCUPwrDwnAllow : Outport  Port=14
  wires:
  Ground/1 -> MCU1_TMSpeed/1
  Ground1/1 -> MCU1_ActTMTorque/1
  Ground2/1 -> MCU1_TMCapacitanceVoltage/1
  Ground3/1 -> MCU1_ActualTMTorqueValid/1
  Ground4/1 -> MCU1_MCU1 PrechargeAllow/1
  Constant/1 -> MCU1_TMStatus/1
  Ground6/1 -> MCU1_TMErrorStatus/1
  Ground7/1 -> MCU1_TM MAMTorque/1
  Ground8/1 -> MCU1_TM MAGTorque/1
  Ground9/1 -> MCU1_CalTMTorque/1
  Ground10/1 -> MCU1_CoolingRequest/1
  Ground11/1 -> PWM_Status/1
  Ground12/1 -> EM_trq_req/1
  In1/1 -> Terminator/1
  Constant11/1 -> bool_MCUPwrDwnAllow/1

== system HQEV_MiL_20160830_integrate_2010a/MiL/Test_Integration/MCU_FF/MCU/MCU/Standby/Subsystem ==
  In1 : Inport
  Bus Selector1 : BusSelector  OutputSignals=Motor_F.EM1_spd
  Bus Selector2 : BusSelector  OutputSignals=Motor_F.EM1_U
  Constant{,1,3..7,9..10} (9 alike) : Constant  Value=0
  Constant11 : Constant
  Constant2 : Constant  Value=2
  Subsystem : Subsystem
  Unit Delay : UnitDelay  SampleTime=-1
  Unit Delay1 : UnitDelay  SampleTime=-1
  MCU1_TMSpeed : Outport
  MCU1_ActTMTorque : Outport  Port=2
  MCU1_TMCapacitanceVoltage : Outport  Port=3
  MCU1_ActualTMTorqueValid : Outport  Port=4
  MCU1_MCU1 PrechargeAllow : Outport  Port=5
  MCU1_TMStatus : Outport  Port=6
  MCU1_TMErrorStatus : Outport  Port=7
  MCU1_TM MAMTorque : Outport  Port=8
  MCU1_TM MAGTorque : Outport  Port=9
  MCU1_CalTMTorque : Outport  Port=10
  MCU1_CoolingRequest : Outport  Port=11
  PWM_Status : Outport  Port=12
  EM_trq_req : Outport  Port=13
  bool_MCUPwrDwnAllow : Outport  Port=14
  wires:
  Constant10/1 -> MCU1_ActTMTorque/1
  Constant/1 -> MCU1_ActualTMTorqueValid/1
  Constant1/1 -> MCU1_MCU1 PrechargeAllow/1
  Constant2/1 -> MCU1_TMStatus/1
  Constant3/1 -> MCU1_TMErrorStatus/1
  Constant4/1 -> MCU1_TM MAMTorque/1
  Constant5/1 -> MCU1_TM MAGTorque/1
  Constant6/1 -> MCU1_CalTMTorque/1
  Constant7/1 -> MCU1_CoolingRequest/1
  Subsystem/1(PWM) -> PWM_Status/1
  Constant9/1 -> EM_trq_req/1
  In1/1 -> Bus Selector1/1, Bus Selector2/1
  Bus Selector2/1 -> Unit Delay1/1  "<EM1_U>"
  Bus Selector1/1 -> Unit Delay/1  "<EM1_spd>"
  Unit Delay/1 -> MCU1_TMSpeed/1, Subsystem/1(EM_spd)
  Unit Delay1/1 -> MCU1_TMCapacitanceVoltage/1
  Constant11/1 -> bool_MCUPwrDwnAllow/1

== system HQEV_MiL_20160830_integrate_2010a/MiL/Test_Integration/MCU_FF/MCU/MCU/Stop/Subsystem ==
  In1 : Inport
  Bus Selector : BusSelector  OutputSignals=Motor_F.EM1_spd
  Bus Selector1 : BusSelector  OutputSignals=Motor_F.EM1_U
  Constant{,3..7,9..10} (8 alike) : Constant  Value=0
  Constant1 : Constant
  Constant11 : Constant
  Constant2 : Constant  Value=4
  Subsystem : Subsystem
  Unit Delay : UnitDelay  SampleTime=-1
  Unit Delay1 : UnitDelay  SampleTime=-1
  MCU1_TMSpeed : Outport
  MCU1_ActTMTorque : Outport  Port=2
  MCU1_TMCapacitanceVoltage : Outport  Port=3
  MCU1_ActualTMTorqueValid : Outport  Port=4
  MCU1_MCU1 PrechargeAllow : Outport  Port=5
  MCU1_TMStatus : Outport  Port=6
  MCU1_TMErrorStatus : Outport  Port=7
  MCU1_TM MAMTorque : Outport  Port=8
  MCU1_TM MAGTorque : Outport  Port=9
  MCU1_CalTMTorque : Outport  Port=10
  MCU1_CoolingRequest : Outport  Port=11
  PWM_Status : Outport  Port=12
  EM_trq_req : Outport  Port=13
  bool_MCUPwrDwnAllow : Outport  Port=14
  wires:
  Constant10/1 -> MCU1_ActTMTorque/1
  Constant/1 -> MCU1_ActualTMTorqueValid/1
  Constant1/1 -> MCU1_MCU1 PrechargeAllow/1
  Constant2/1 -> MCU1_TMStatus/1
  Constant3/1 -> MCU1_TMErrorStatus/1
  Constant4/1 -> MCU1_TM MAMTorque/1
  Constant5/1 -> MCU1_TM MAGTorque/1
  Constant6/1 -> MCU1_CalTMTorque/1
  Constant7/1 -> MCU1_CoolingRequest/1
  Constant9/1 -> EM_trq_req/1
  Subsystem/1(PWM) -> PWM_Status/1
  Bus Selector/1 -> Unit Delay/1  "<EM1_spd>"
  Bus Selector1/1 -> Unit Delay1/1  "<EM1_U>"
  In1/1 -> Bus Selector/1, Bus Selector1/1
  Unit Delay/1 -> MCU1_TMSpeed/1, Subsystem/1(EM_spd)
  Unit Delay1/1 -> MCU1_TMCapacitanceVoltage/1
  Constant11/1 -> bool_MCUPwrDwnAllow/1

== system HQEV_MiL_20160830_integrate_2010a/MiL/Test_Integration/MCU_FF/MCU/MCU/Torque_Control/Subsystem ==
  In1 : Inport
  Bus Selector : BusSelector  OutputSignals=Motor_F.EM1_spd,Motor_F.EM1_trq_out,Motor_F.EM1_U,HCU.HCU_TMTorqueRequestToMCU1
  Constant : Constant
  Constant1 : Constant
  Constant11 : Constant  Value=0
  Constant2 : Constant  Value=3
  Constant3 : Constant  Value=0
  Constant4 : Constant  Value=0
  Constant5 : Constant
  Constant6 : Constant  Value=300
  Data Type Conversion4 : DataTypeConversion  OutDataTypeMode=double  OutDataTypeStr=double
  Max_Torque : Subsystem  TreatAsAtomicUnit=on
  Unit Delay{,1..3} (4 alike) : UnitDelay  SampleTime=-1
  MCU1_TMSpeed : Outport
  MCU1_ActTMTorque : Outport  Port=2
  MCU1_TMCapacitanceVoltage : Outport  Port=3
  MCU1_ActualTMTorqueValid : Outport  Port=4
  MCU1_MCU1 PrechargeAllow : Outport  Port=5
  MCU1_TMStatus : Outport  Port=6
  MCU1_TMErrorStatus : Outport  Port=7
  MCU1_TM MAMTorque : Outport  Port=8
  MCU1_TM MAGTorque : Outport  Port=9
  MCU1_CalTMTorque : Outport  Port=10
  MCU1_CoolingRequest : Outport  Port=11
  PWM_Status : Outport  Port=12
  EM_trq_req : Outport  Port=13
  bool_MCUPwrDwnAllow : Outport  Port=14
  wires:
  Max_Torque/1(Max_Mot_Torque) -> MCU1_TM MAMTorque/1
  Max_Torque/2(Max_Gen_Torque) -> MCU1_TM MAGTorque/1
  Constant/1 -> MCU1_ActualTMTorqueValid/1
  Constant1/1 -> MCU1_MCU1 PrechargeAllow/1
  Constant2/1 -> MCU1_TMStatus/1
  Constant3/1 -> MCU1_TMErrorStatus/1
  Constant4/1 -> MCU1_CoolingRequest/1
  Constant5/1 -> PWM_Status/1
  In1/1 -> Bus Selector/1
  Bus Selector/1 -> Max_Torque/2(EM_spd), Unit Delay/1  "<EM1_spd>"
  Bus Selector/2 -> Unit Delay1/1, Unit Delay3/1  "<EM1_trq_out>"
  Bus Selector/3 -> Unit Delay2/1  "<EM1_U>"
  Constant6/1 -> Max_Torque/1(EM_Volt)
  Data Type Conversion4/1 -> EM_trq_req/1
  Bus Selector/4 -> Data Type Conversion4/1  "<HCU_TMTorqueRequestToMCU1>"
  Unit Delay/1 -> MCU1_TMSpeed/1
  Unit Delay1/1 -> MCU1_ActTMTorque/1
  Unit Delay2/1 -> MCU1_TMCapacitanceVoltage/1
  Unit Delay3/1 -> MCU1_CalTMTorque/1
  Constant11/1 -> bool_MCUPwrDwnAllow/1

== system HQEV_MiL_20160830_integrate_2010a/MiL/Test_Integration/MCU_RR/MCU/MCU/Subsystem14/GSD ==
  In1 : Inport
  function : TriggerPort  TriggerType=function-call
  Bus Creator : BusCreator  Inputs=14
  Subsystem : Subsystem
  Out1 : Outport
  wires:
  Subsystem/13(EM_trq_req) -> Bus Creator/13
  Subsystem/12(PWM_Status) -> Bus Creator/12
  Subsystem/11(MCU1_CoolingRequest) -> Bus Creator/11
  Subsystem/10(MCU1_CalTMTorque) -> Bus Creator/10
  Subsystem/9(MCU1_TM MAGTorque) -> Bus Creator/9
  Subsystem/8(MCU1_TM MAMTorque) -> Bus Creator/8
  Subsystem/7(MCU1_TMErrorStatus) -> Bus Creator/7
  Subsystem/6(MCU1_TMStatus) -> Bus Creator/6
  Subsystem/5(MCU1_MCU1 PrechargeAllow) -> Bus Creator/5
  Subsystem/4(MCU1_ActualTMTorqueValid) -> Bus Creator/4
  Subsystem/3(MCU1_TMCapacitanceVoltage) -> Bus Creator/3
  Subsystem/2(MCU1_ActTMTorque) -> Bus Creator/2
  Subsystem/1(MCU1_TMSpeed) -> Bus Creator/1
  Bus Creator/1 -> Out1/1
  In1/1 -> Subsystem/1(In1)
  Subsystem/14(bool_MCUPwrDwnAllow) -> Bus Creator/14

== system HQEV_MiL_20160830_integrate_2010a/MiL/Test_Integration/MCU_RR/MCU/MCU/Subsystem14/Init ==
  In1 : Inport
  function : TriggerPort  TriggerType=function-call
  Bus Creator : BusCreator  Inputs=14
  Subsystem : Subsystem
  Out1 : Outport
  wires:
  Bus Creator/1 -> Out1/1
  Subsystem/13(EM2_trq_req) -> Bus Creator/13
  Subsystem/12(PWM_Status) -> Bus Creator/12
  Subsystem/11(MCU2_CoolingRequest) -> Bus Creator/11
  Subsystem/10(MCU2_CalTMTorque) -> Bus Creator/10
  Subsystem/9(MCU2_TM MAGTorque) -> Bus Creator/9
  Subsystem/8(MCU2_TM MAMTorque) -> Bus Creator/8
  Subsystem/7(MCU2_TMErrorStatus) -> Bus Creator/7
  Subsystem/6(MCU2_TMStatus) -> Bus Creator/6
  Subsystem/5(MCU2_PrechargeAllow) -> Bus Creator/5
  Subsystem/4(MCU2_ActualTMTorqueValid) -> Bus Creator/4
  Subsystem/3(MCU2_TMCapacitanceVoltage) -> Bus Creator/3
  Subsystem/2(MCU2_ActTMTorque) -> Bus Creator/2
  Subsystem/1(MCU2_TMSpeed) -> Bus Creator/1
  In1/1 -> Subsystem/1(In1)
  Subsystem/14(bool_MCUPwrDwnAllow) -> Bus Creator/14

== system HQEV_MiL_20160830_integrate_2010a/MiL/Test_Integration/MCU_RR/MCU/MCU/Subsystem14/Invalid ==
  In1 : Inport
  function : TriggerPort  TriggerType=function-call
  Bus Creator : BusCreator  Inputs=14
  Subsystem : Subsystem
  Out1 : Outport
  wires:
  Subsystem/13(EM_trq_req) -> Bus Creator/13
  Subsystem/12(PWM_Status) -> Bus Creator/12
  Subsystem/11(MCU1_CoolingRequest) -> Bus Creator/11
  Subsystem/10(MCU1_CalTMTorque) -> Bus Creator/10
  Subsystem/9(MCU1_TM MAGTorque) -> Bus Creator/9
  Subsystem/8(MCU1_TM MAMTorque) -> Bus Creator/8
  Subsystem/7(MCU1_TMErrorStatus) -> Bus Creator/7
  Subsystem/6(MCU1_TMStatus) -> Bus Creator/6
  Subsystem/5(MCU1_MCU1 PrechargeAllow) -> Bus Creator/5
  Subsystem/4(MCU1_ActualTMTorqueValid) -> Bus Creator/4
  Subsystem/3(MCU1_TMCapacitanceVoltage) -> Bus Creator/3
  Subsystem/2(MCU1_ActTMTorque) -> Bus Creator/2
  Subsystem/1(MCU1_TMSpeed) -> Bus Creator/1
  Bus Creator/1 -> Out1/1
  In1/1 -> Subsystem/1(In1)
  Subsystem/14(bool_MCUPwrDwnAllow) -> Bus Creator/14

== system HQEV_MiL_20160830_integrate_2010a/MiL/Test_Integration/MCU_RR/MCU/MCU/Subsystem14/Precharge ==
  In1 : Inport
  function : TriggerPort  TriggerType=function-call
  Bus Creator : BusCreator  Inputs=14
  Subsystem : Subsystem
  Out1 : Outport
  wires:
  In1/1 -> Subsystem/1(In1)
  Bus Creator/1 -> Out1/1
  Subsystem/12(PWM_Status) -> Bus Creator/12
  Subsystem/6(MCU1_TMStatus) -> Bus Creator/6
  Subsystem/11(MCU1_CoolingRequest) -> Bus Creator/11
  Subsystem/5(MCU1_MCU1 PrechargeAllow) -> Bus Creator/5
  Subsystem/10(MCU1_CalTMTorque) -> Bus Creator/10
  Subsystem/9(MCU1_TM MAGTorque) -> Bus Creator/9
  Subsystem/13(EM_trq_req) -> Bus Creator/13
  Subsystem/3(MCU1_TMCapacitanceVoltage) -> Bus Creator/3
  Subsystem/2(MCU1_ActTMTorque) -> Bus Creator/2
  Subsystem/4(MCU1_ActualTMTorqueValid) -> Bus Creator/4
  Subsystem/1(MCU1_TMSpeed) -> Bus Creator/1
  Subsystem/8(MCU1_TM MAMTorque) -> Bus Creator/8
  Subsystem/7(MCU1_TMErrorStatus) -> Bus Creator/7
  Subsystem/14(bool_MCUPwrDwnAllow) -> Bus Creator/14

== system HQEV_MiL_20160830_integrate_2010a/MiL/Test_Integration/MCU_RR/MCU/MCU/Subsystem14/Rapid_Discharge ==
  In1 : Inport
  function : TriggerPort  TriggerType=function-call
  Bus Creator : BusCreator  Inputs=14
  Subsystem : Subsystem
  Out1 : Outport
  wires:
  Bus Creator/1 -> Out1/1
  In1/1 -> Subsystem/1(In1)
  Subsystem/13(EM_trq_req) -> Bus Creator/13
  Subsystem/12(PWM_Status) -> Bus Creator/12
  Subsystem/2(MCU1_ActTMTorque) -> Bus Creator/2
  Subsystem/4(MCU1_ActualTMTorqueValid) -> Bus Creator/4
  Subsystem/11(MCU1_CoolingRequest) -> Bus Creator/11
  Subsystem/3(MCU1_TMCapacitanceVoltage) -> Bus Creator/3
  Subsystem/9(MCU1_TM MAGTorque) -> Bus Creator/9
  Subsystem/7(MCU1_TMErrorStatus) -> Bus Creator/7
  Subsystem/8(MCU1_TM MAMTorque) -> Bus Creator/8
  Subsystem/10(MCU1_CalTMTorque) -> Bus Creator/10
  Subsystem/5(MCU1_MCU1 PrechargeAllow) -> Bus Creator/5
  Subsystem/6(MCU1_TMStatus) -> Bus Creator/6
  Subsystem/1(MCU1_TMSpeed) -> Bus Creator/1
  Subsystem/14(bool_MCUPwrDwnAllow) -> Bus Creator/14

== system HQEV_MiL_20160830_integrate_2010a/MiL/Test_Integration/MCU_RR/MCU/MCU/Subsystem14/Sleep ==
  In1 : Inport
  function : TriggerPort  TriggerType=function-call
  Bus Creator : BusCreator  Inputs=14
  Subsystem : Subsystem
  Out1 : Outport
  wires:
  Subsystem/13(EM_trq_req) -> Bus Creator/13
  Subsystem/12(PWM_Status) -> Bus Creator/12
  Subsystem/11(MCU1_CoolingRequest) -> Bus Creator/11
  Subsystem/10(MCU1_CalTMTorque) -> Bus Creator/10
  Subsystem/9(MCU1_TM MAGTorque) -> Bus Creator/9
  Subsystem/8(MCU1_TM MAMTorque) -> Bus Creator/8
  Subsystem/7(MCU1_TMErrorStatus) -> Bus Creator/7
  Subsystem/6(MCU1_TMStatus) -> Bus Creator/6
  Subsystem/5(MCU1_MCU1 PrechargeAllow) -> Bus Creator/5
  Subsystem/4(MCU1_ActualTMTorqueValid) -> Bus Creator/4
  Subsystem/3(MCU1_TMCapacitanceVoltage) -> Bus Creator/3
  Subsystem/2(MCU1_ActTMTorque) -> Bus Creator/2
  Subsystem/1(MCU1_TMSpeed) -> Bus Creator/1
  Bus Creator/1 -> Out1/1
  In1/1 -> Subsystem/1(In1)
  Subsystem/14(bool_MCUPwrDwnAllow) -> Bus Creator/14

== system HQEV_MiL_20160830_integrate_2010a/MiL/Test_Integration/MCU_RR/MCU/MCU/Subsystem14/Standby ==
  In1 : Inport
  function : TriggerPort  TriggerType=function-call
  Bus Creator : BusCreator  Inputs=14
  Subsystem : Subsystem
  Out1 : Outport
  wires:
  In1/1 -> Subsystem/1(In1)
  Bus Creator/1 -> Out1/1
  Subsystem/5(MCU1_MCU1 PrechargeAllow) -> Bus Creator/5
  Subsystem/10(MCU1_CalTMTorque) -> Bus Creator/10
  Subsystem/7(MCU1_TMErrorStatus) -> Bus Creator/7
  Subsystem/13(EM_trq_req) -> Bus Creator/13
  Subsystem/4(MCU1_ActualTMTorqueValid) -> Bus Creator/4
  Subsystem/11(MCU1_CoolingRequest) -> Bus Creator/11
  Subsystem/8(MCU1_TM MAMTorque) -> Bus Creator/8
  Subsystem/2(MCU1_ActTMTorque) -> Bus Creator/2
  Subsystem/1(MCU1_TMSpeed) -> Bus Creator/1
  Subsystem/12(PWM_Status) -> Bus Creator/12
  Subsystem/3(MCU1_TMCapacitanceVoltage) -> Bus Creator/3
  Subsystem/6(MCU1_TMStatus) -> Bus Creator/6
  Subsystem/9(MCU1_TM MAGTorque) -> Bus Creator/9
  Subsystem/14(bool_MCUPwrDwnAllow) -> Bus Creator/14

== system HQEV_MiL_20160830_integrate_2010a/MiL/Test_Integration/MCU_RR/MCU/MCU/Subsystem14/Stop ==
  In1 : Inport
  function : TriggerPort  TriggerType=function-call
  Bus Creator : BusCreator  Inputs=14
  Subsystem : Subsystem
  Out1 : Outport
  wires:
  In1/1 -> Subsystem/1(In1)
  Subsystem/13(EM_trq_req) -> Bus Creator/13
  Subsystem/12(PWM_Status) -> Bus Creator/12
  Subsystem/11(MCU1_CoolingRequest) -> Bus Creator/11
  Subsystem/10(MCU1_CalTMTorque) -> Bus Creator/10
  Subsystem/9(MCU1_TM MAGTorque) -> Bus Creator/9
  Subsystem/8(MCU1_TM MAMTorque) -> Bus Creator/8
  Subsystem/7(MCU1_TMErrorStatus) -> Bus Creator/7
  Subsystem/6(MCU1_TMStatus) -> Bus Creator/6
  Subsystem/5(MCU1_MCU1 PrechargeAllow) -> Bus Creator/5
  Subsystem/4(MCU1_ActualTMTorqueValid) -> Bus Creator/4
  Subsystem/3(MCU1_TMCapacitanceVoltage) -> Bus Creator/3
  Subsystem/2(MCU1_ActTMTorque) -> Bus Creator/2
  Subsystem/1(MCU1_TMSpeed) -> Bus Creator/1
  Bus Creator/1 -> Out1/1
  Subsystem/14(bool_MCUPwrDwnAllow) -> Bus Creator/14

== system HQEV_MiL_20160830_integrate_2010a/MiL/Test_Integration/MCU_RR/MCU/MCU/Subsystem14/Torque_Control ==
  In1 : Inport
  function : TriggerPort  TriggerType=function-call
  Bus Creator : BusCreator  Inputs=14
  Subsystem : Subsystem
  Out1 : Outport
  wires:
  In1/1 -> Subsystem/1(In1)
  Bus Creator/1 -> Out1/1
  Subsystem/13(EM_trq_req) -> Bus Creator/13
  Subsystem/9(MCU1_TM MAGTorque) -> Bus Creator/9
  Subsystem/1(MCU1_TMSpeed) -> Bus Creator/1
  Subsystem/11(MCU1_CoolingRequest) -> Bus Creator/11
  Subsystem/4(MCU1_ActualTMTorqueValid) -> Bus Creator/4
  Subsystem/12(PWM_Status) -> Bus Creator/12
  Subsystem/2(MCU1_ActTMTorque) -> Bus Creator/2
  Subsystem/3(MCU1_TMCapacitanceVoltage) -> Bus Creator/3
  Subsystem/8(MCU1_TM MAMTorque) -> Bus Creator/8
  Subsystem/10(MCU1_CalTMTorque) -> Bus Creator/10
  Subsystem/5(MCU1_MCU1 PrechargeAllow) -> Bus Creator/5
  Subsystem/7(MCU1_TMErrorStatus) -> Bus Creator/7
  Subsystem/6(MCU1_TMStatus) -> Bus Creator/6
  Subsystem/14(bool_MCUPwrDwnAllow) -> Bus Creator/14

== system HQEV_MiL_20160830_integrate_2010a/MiL/Test_Integration/Motor_FF/Motor/Motor/Uc_Management/Open ==
  RapidDischargeEnable : Inport
  Uc : Inport  Port=2
  Bus Creator : BusCreator  Inputs=2
  Constant : Constant  Value=1.0000e-006
  Constant1 : Constant  Value=0
  EM_C : Constant  Value=600
      settings: AttributesFormatString=Unit:muF
  F : Product  RndMeth=Zero
  RC : Product  RndMeth=Zero
  R_precharge : Constant  Value=1000
      settings: AttributesFormatString=Unit:ohm
  Switch : Switch  Criteria=u2 ~= 0
  Out1 : Outport
  wires:
  EM_C/1 -> F/1
  Constant/1 -> F/2
  R_precharge/1 -> RC/1
  F/1 -> RC/2
  RC/1 -> Bus Creator/2  "RC"
  RapidDischargeEnable/1 -> Switch/2
  Uc/1 -> Switch/3
  Switch/1 -> Bus Creator/1  "U_Term"
  Constant1/1 -> Switch/1
  Bus Creator/1 -> Out1/1

== system HQEV_MiL_20160830_integrate_2010a/MiL/Test_Integration/Motor_FF/Motor/Motor/Uc_Management/PreCharg ==
  Bat_U : Inport
  Bus Creator : BusCreator  Inputs=2
  Constant : Constant  Value=1.0000e-006
  EM_C : Constant  Value=600
      settings: AttributesFormatString=Unit:muF
  F : Product  RndMeth=Zero
  RC : Product  RndMeth=Zero
  R_precharge : Constant  Value=55
      settings: AttributesFormatString=Unit:ohm
  Out : Outport
  wires:
  Bus Creator/1 -> Out/1
  Bat_U/1 -> Bus Creator/1  "U_Term"
  EM_C/1 -> F/1
  Constant/1 -> F/2
  R_precharge/1 -> RC/1
  F/1 -> RC/2
  RC/1 -> Bus Creator/2  "RC"
